simulink model "simulation"  (R2016a)
settings: Solver=VariableStepAuto  StartTime=0.0  StopTime=10.0  RelTol=1e-3
libraries: powerlib x10, powerlib_meascontrol x6
settings Model: Creator=Hakan Polat  LastModifiedBy=Hakan Polat

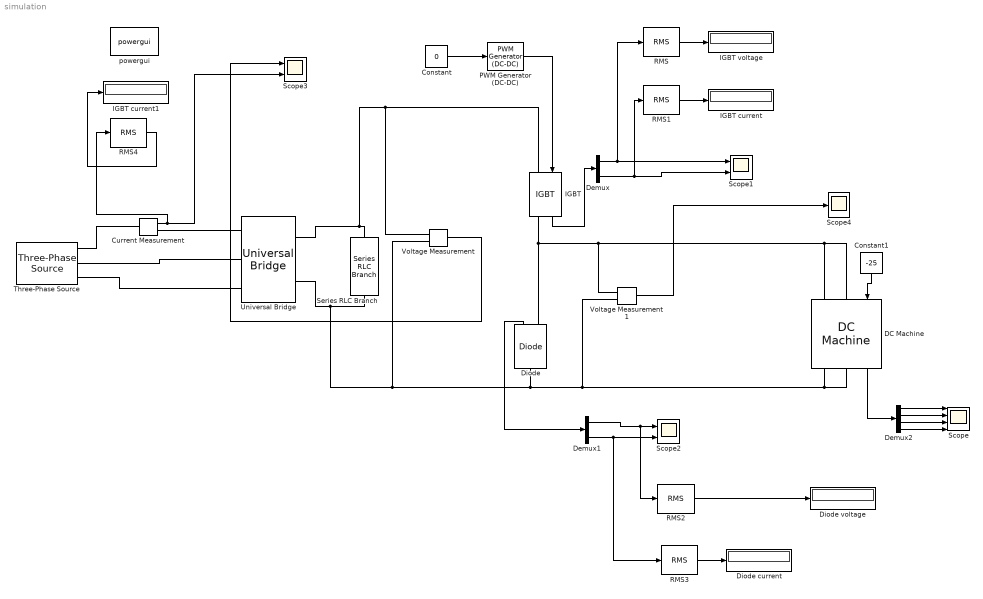
== system simulation ==
  Constant : Constant  Value=0
  Constant1 : Constant  Value=-25
  Current Measurement : powerlib/Measurements/Current Measurement  PhasorSimulation=off  OutputType=Complex  PSBequivalent=0
  DC Machine : powerlib/Machines/DC Machine  PresetModel=No  MechanicalLoad=Torque TL  FieldType=Wound  ShowDetailedParameters=on  MeasurementBus=off  RLa="[ 28  0.0133]"  RLf="[ 8260  6.4]"  Laf=1.8  MachineConstant=Torque constant (N.m/A)  Ke=1.8  Kt=1.8  J=1  Bm=0  Tf=0  w0=1  Ifinit=1  TsPowergui=0  TsBlock=-1
  Demux : Demux  Outputs=2
  Demux1 : Demux  Outputs=2
  Demux2 : Demux
  Diode : powerlib/Power Electronics/Diode  Ron=0.001  Lon=0  Vf=0.8  IC=0  UseSnubber=off  Rs=500  Cs=250e-9  Measurements=on
  Diode current : Display
  Diode voltage : Display
  IGBT : powerlib/Power Electronics/IGBT  Ron=0.001  Lon=0  Vf=1  Tf=1e-6  Tt=2e-6  IC=0  Rs=1e5  Cs=inf  Measurements=on
  IGBT current : Display
  IGBT current1 : Display
  IGBT voltage : Display
  PWM Generator (DC-DC) : powerlib_meascontrol/Pulse & Signal Generators/PWM Generator (DC-DC)  Fsw=3900  Ts=0
  RMS{,1..3} (4 alike) : powerlib_meascontrol/Measurements/RMS  TrueRMS=on  Freq=3900  RMSInit=120  Ts=0
  RMS4 : powerlib_meascontrol/Measurements/RMS  TrueRMS=on  Freq=50  RMSInit=120  Ts=0
  Scope : Scope  NumInputPorts=4
  Scope1 : Scope  NumInputPorts=2
  Scope2 : Scope  NumInputPorts=2
  Scope3 : Scope  NumInputPorts=2
  Scope4 : Scope
  Series RLC Branch : powerlib/Elements/Series RLC Branch  LConnTagsString=__new0  RConnTagsString=__new0  BranchType=C  Resistance=1  Inductance=1e-3  SetiL0=off  InitialCurrent=0  Capacitance=680e-6  Setx0=off  InitialVoltage=0  Measurements=None
  Three-Phase Source : powerlib/Electrical Sources/Three-Phase Source  InternalConnection=Yg  VoltagePhases=off  Voltage=160  PhaseAngle=0  Voltage_phases=[25e3 25e3 25e3]/sqrt(3)  PhaseAngles_phases=[0 -120 +120]  Frequency=50  NonIdealSource=on  SpecifyImpedance=off  Resistance=0  Inductance=0  ShortCircuitLevel=100e6  BaseVoltage=0  XRratio=7  BusType=swing  Pref=10e3  Qref=0  Prefabc=[10e3, 10e3, 10e3]  Qrefabc=[0, 0, 0]  Qmin=-inf  Qmax=inf
  Universal Bridge : powerlib/Power Electronics/Universal Bridge  Arms=3  SnubberResistance=1e5  SnubberCapacitance=inf  Device=Diodes  Ron=1e-3  Lon=0  ForwardVoltages="[  0  0  ]"  ForwardVoltage=0  GTOparameters=[ 10e-6 , 20e-6 ]  IGBTparameters=[ 1e-6 , 2e-6 ]  Measurements=None  Measurements_2=None  converterType=Rectifier
  Voltage Measurement : powerlib/Measurements/Voltage Measurement  PhasorSimulation=off  OutputType=Complex  PSBequivalent=0
  Voltage Measurement1 : powerlib/Measurements/Voltage Measurement  PhasorSimulation=off  OutputType=Complex  PSBequivalent=0
  powergui : powerlib/powergui  Priority=1  SimulationMode=Continuous  SolverType=Tustin/Backward Euler (TBE)  SampleTime=50e-6  frequency=60  SPID=off  DisableSnubberDevices=off  DisableRonSwitches=off  DisableVfSwitches=off  SwTol=0  DisplayEquations=off  Interpol=off  ExternalGateDelay=off  methode=off  Ts=10  FunctionMessages=off  echomessages=off  HookPort=off  EnableUseOfTLC=off  x0status=blocks  frequencyindice=0  Pbase=100e6  ErrMax=1e-4  Iterations=50  UnitsV=kV  UnitsW=MW  buscounter=0  RestoreLinks=warning  ResistiveCurrentMeasurement=off  Frange=[0:2:500]  Ylog=off  Xlog=on  ShowGrid=off  save=off  variable=ZData  structure=0  ZoomFFT=off  StartTime=0.0  cycles=1  DisplayStyle=1  fundamental=60  FreqAxis=off  MaxFrequency=1000  frequencyindicesteady=1  RmsSteady=1  display=off
  wires:
  PWM Generator (DC-DC)/1 -> IGBT/1
  Constant/1 -> PWM Generator (DC-DC)/1
  Constant1/1 -> DC Machine/1
  IGBT/1 -> Demux/1
  Diode/1 -> Demux1/1
  DC Machine/1 -> Demux2/1
  Demux/1 -> RMS/1, Scope1/1
  Demux/2 -> RMS1/1, Scope1/2
  Demux1/2 -> RMS3/1, Scope2/2
  Demux1/1 -> RMS2/1, Scope2/1
  Demux2/1 -> Scope/1
  Demux2/2 -> Scope/2
  Demux2/3 -> Scope/3
  Demux2/4 -> Scope/4
  RMS/1 -> IGBT voltage/1
  RMS1/1 -> IGBT current/1
  RMS3/1 -> Diode current/1
  Voltage Measurement/1 -> Scope3/1
  Voltage Measurement1/1 -> Scope4/1
  RMS2/1 -> Diode voltage/1
  Current Measurement/1 -> Scope3/2, RMS4/1
  RMS4/1 -> IGBT current1/1
  connections:
  Universal Bridge/LConn2 -- Three-Phase Source/RConn2
  Universal Bridge/LConn3 -- Three-Phase Source/RConn3
  Universal Bridge/RConn1 -- Voltage Measurement/LConn1 -- IGBT/LConn1 -- Series RLC Branch/LConn1
  Universal Bridge/RConn2 -- Voltage Measurement/LConn2 -- DC Machine/RConn2 -- DC Machine/RConn1 -- Voltage Measurement1/LConn2 -- Diode/LConn1 -- Series RLC Branch/RConn1
  IGBT/RConn1 -- DC Machine/LConn2 -- DC Machine/LConn1 -- Voltage Measurement1/LConn1 -- Diode/RConn1
  Current Measurement/RConn1 -- Universal Bridge/LConn1
  Current Measurement/LConn1 -- Three-Phase Source/RConn1
